simulink model "FP667_Jerrar_Bukhari_Luenberger_nonlinear"  (R2017b)
settings: Solver=FixedStepAuto  StartTime=0.0  StopTime=60  FixedStep=0.05  RelTol=1e-3
values from neighbouring files (symbols this model uses):
  A = [0 1 0 0 0 0 ... (first row only)    [ENPM667FinalProject_JerrarBukhari_MatlabCode.m]
  B = [ 0 ... (first row only)    [ENPM667FinalProject_JerrarBukhari_MatlabCode.m]
  C = [ 1 0 0 0 0 0 ... (first row only)    [ENPM667FinalProject_JerrarBukhari_MatlabCode.m]
  g = 9.8    [ENPM667FinalProject_JerrarBukhari_MatlabCode.m]
  L = place(A',C',P)'    [ENPM667FinalProject_JerrarBukhari_MatlabCode.m]
  l1 = 20    [ENPM667FinalProject_JerrarBukhari_MatlabCode.m]
  l2 = 10    [ENPM667FinalProject_JerrarBukhari_MatlabCode.m]
  M = 1000    [ENPM667FinalProject_JerrarBukhari_MatlabCode.m]
  m1 = 100    [ENPM667FinalProject_JerrarBukhari_MatlabCode.m]
  m2 = 100    [ENPM667FinalProject_JerrarBukhari_MatlabCode.m]
undefined symbols (not defined in the file or in its folder): K
settings Model: Creator=Jerrar  LastModifiedBy=Jerrar

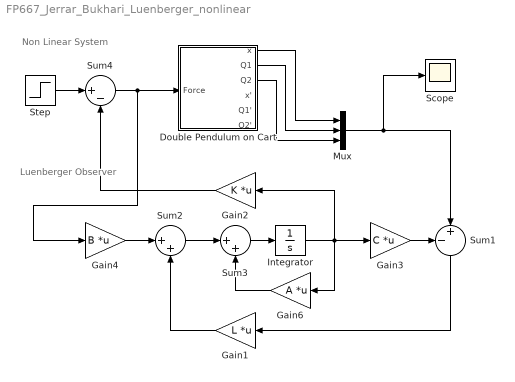
== system FP667_Jerrar_Bukhari_Luenberger_nonlinear ==
  note: Non Linear System
  note: Luenberger
      |  Observer
  Double Pendulum on Cart : Subsystem
  Gain1 : Gain  Gain=L  Multiplication=Matrix(K*u)
  Gain2 : Gain  Gain=K  Multiplication=Matrix(K*u)
  Gain3 : Gain  Gain=C  Multiplication=Matrix(K*u)
  Gain4 : Gain  Gain=B  Multiplication=Matrix(K*u)
  Gain6 : Gain  Gain=A  Multiplication=Matrix(K*u)
  Integrator : Integrator
  Mux : Mux  Inputs=3
  Scope : Scope
  Step : Step  SampleTime=0
  Sum1 : Sum  Inputs=-+|
  Sum2 : Sum  Inputs=|++
  Sum3 : Sum  Inputs=|++
  Sum4 : Sum  Inputs=|+-
  wires:
  Gain1/1 -> Sum2/2
  Gain4/1 -> Sum2/1
  Integrator/1 -> Gain2/1, Gain6/1, Gain3/1
  Sum2/1 -> Sum3/1
  Gain6/1 -> Sum3/2
  Sum3/1 -> Integrator/1
  Gain2/1 -> Sum4/2
  Step/1 -> Sum4/1
  Sum4/1 -> Double Pendulum on Cart/1(Force), Gain4/1
  Gain3/1 -> Sum1/1
  Sum1/1 -> Gain1/1
  Mux/1 -> Sum1/2, Scope/1
  Double Pendulum on Cart/1(x) -> Mux/1
  Double Pendulum on Cart/2(Q1) -> Mux/2
  Double Pendulum on Cart/3(Q2) -> Mux/3

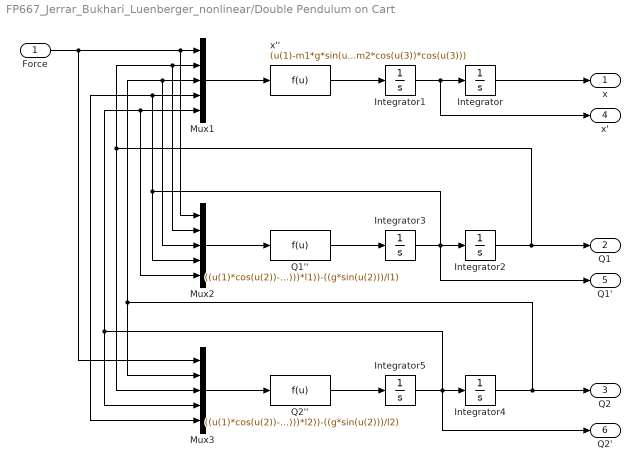
== system FP667_Jerrar_Bukhari_Luenberger_nonlinear/Double Pendulum on Cart ==
  Force : Inport
  Integrator{,1..5} (6 alike) : Integrator
  Mux1 : Mux  Inputs=5
  Mux2 : Mux  Inputs=5
  Mux3 : Mux  Inputs=5
  Q1'' : Fcn  Expr=((u(1)*cos(u(2))-m1*g*sin(u(2))*cos(u(2))*cos(u(2))-m1*l1*(u(4)^2)*sin(u(2))*cos(u(2))-m2*g*sin(u(3))*cos(u(3))*cos(u(2))-m2*l2*(u(5)^2)*sin(u(3))*cos(u(2)))/((M+m1+m2-m1*cos(u(2))*cos(u(2))-m2*cos(u(3))*cos(u(3)))*l1))-((g*sin(u(2)))/l1)
  Q2'' : Fcn  Expr=((u(1)*cos(u(2))-m1*g*sin(u(2))*cos(u(2))*cos(u(2))-m1*l1*(u(4)^2)*sin(u(2))*cos(u(2))-m2*g*sin(u(3))*cos(u(3))*cos(u(2))-m2*l2*(u(5)^2)*sin(u(3))*cos(u(2)))/((M+m1+m2-m1*cos(u(2))*cos(u(2))-m2*cos(u(3))*cos(u(3)))*l2))-((g*sin(u(2)))/l2)
  x'' : Fcn  Expr=(u(1)-m1*g*sin(u(2))*cos(u(2))-m1*l1*(u(4)^2)*sin(u(2))-m2*g*sin(u(3))*cos(u(3))-m2*l2*(u(5)^2)*sin(u(3)))/(M+m1+m2-m1*cos(u(2))*cos(u(2))-m2*cos(u(3))*cos(u(3)))
  x : Outport
  Q1 : Outport  Port=2
  Q2 : Outport  Port=3
  x' : Outport  Port=4
  Q1' : Outport  Port=5
  Q2' : Outport  Port=6
  wires:
  Integrator4/1 -> Q2/1, Mux2/3, Mux1/3, Mux3/2
  Integrator/1 -> x/1
  Mux1/1 -> x''/1
  Integrator3/1 -> Integrator2/1, Mux3/5, Mux1/4, Mux2/4, Q1'/1
  Integrator5/1 -> Q2'/1, Mux3/4, Mux2/5, Mux1/5, Integrator4/1
  Q2''/1 -> Integrator5/1
  Integrator1/1 -> Integrator/1, x'/1
  Force/1 -> Mux2/1, Mux1/1, Mux3/1
  x''/1 -> Integrator1/1
  Integrator2/1 -> Q1/1, Mux2/2, Mux1/2, Mux3/3
  Mux2/1 -> Q1''/1
  Q1''/1 -> Integrator3/1
  Mux3/1 -> Q2''/1
